simulink model "SS_elastico_SP"  (R2024b)
settings: Solver=VariableStepAuto  StartTime=0.0  StopTime=tsamplesimulink  RelTol=1e-3
undefined symbols (not defined in the file): Ac, Bcg, Cc, Dcg, Je, Jm, Kfd, Kfp, Kp, Kv, N, tm
settings Model: Creator=Isaac  LastModifiedBy=ruizh
settings SolverCC: AlgebraicLoopSolver=TrustRegion
settings DataIOCC: ReturnWorkspaceOutputs=off
settings DebuggingCC: UnconnectedInputMsg=warning  UnconnectedOutputMsg=warning  UnconnectedLineMsg=warning  ArithmeticOperatorsInVariantConditions=warning
settings ModelReferenceCC: EnableRefExpFcnMdlSchedulingChecks=on
settings SFSimCC: SimUseLocalCustomCode=off  CustomCodeUndefinedFunction=UseInterfaceOnly
settings RTWCC: RTWUseLocalCustomCode=off  GPUComputeCapability=3.5
settings CodeAppCC: StateflowObjectComments=on

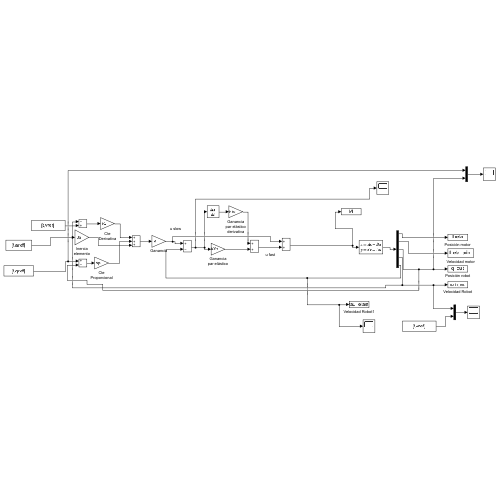
[thumbnail: Simulink's stored preview of the top-level diagram]
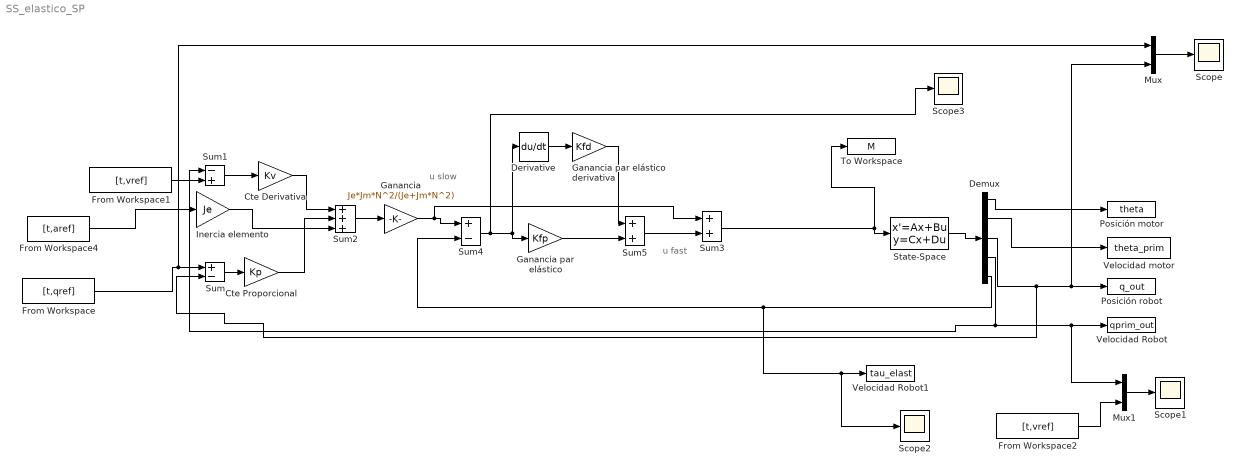
== system SS_elastico_SP ==
  note: u fast
  note: u slow
  Cte Derivativa : Gain  Gain=Kv  SaturateOnIntegerOverflow=on  OutDataTypeStr=Inherit: Same as input  ParamDataTypeStr=Inherit: Same as input
  Cte Proporcional : Gain  Gain=Kp  SaturateOnIntegerOverflow=on  OutDataTypeStr=Inherit: Same as input  ParamDataTypeStr=Inherit: Same as input
  Demux : Demux  Outputs=5
  Derivative : Derivative
  From Workspace : FromWorkspace  VariableName=[t,qref]  SampleTime=tm  ZeroCross=off
  From Workspace1 : FromWorkspace  VariableName=[t,vref]  SampleTime=tm  ZeroCross=off
  From Workspace2 : FromWorkspace  VariableName=[t,vref]  SampleTime=tm  ZeroCross=off
  From Workspace4 : FromWorkspace  VariableName=[t,aref]  SampleTime=tm  ZeroCross=off
  Ganancia : Gain  Gain=Je*Jm*N^2/(Je+Jm*N^2)  SaturateOnIntegerOverflow=on  OutDataTypeStr=Inherit: Same as input  ParamDataTypeStr=Inherit: Same as input
  Ganancia par elástico : Gain  Gain=Kfp  SaturateOnIntegerOverflow=on  OutDataTypeStr=Inherit: Same as input  ParamDataTypeStr=Inherit: Same as input
  Ganancia par elástico derivativa : Gain  Gain=Kfd  SaturateOnIntegerOverflow=on  OutDataTypeStr=Inherit: Same as input  ParamDataTypeStr=Inherit: Same as input
  Inercia elemento : Gain  Gain=Je  SaturateOnIntegerOverflow=on  OutDataTypeStr=Inherit: Same as input  ParamDataTypeStr=Inherit: Same as input
  Mux : Mux  Inputs=2
  Mux1 : Mux  Inputs=2
  Posición motor : ToWorkspace  VariableName=theta  SampleTime=tm
  Posición robot : ToWorkspace  VariableName=q_out  SampleTime=tm
  Scope{,1..3} (4 alike) : Scope
  State-Space : StateSpace  A=Ac  B=Bcg  C=Cc  D=Dcg  InitialCondition=0
  Sum : Sum  Inputs=+-  InputSameDT=on  SaturateOnIntegerOverflow=on  OutDataTypeStr=Inherit: Same as first input
  Sum1 : Sum  Inputs=-+  InputSameDT=on  SaturateOnIntegerOverflow=on  OutDataTypeStr=Inherit: Same as first input
  Sum2 : Sum  Inputs=+++  InputSameDT=on  SaturateOnIntegerOverflow=on  OutDataTypeStr=Inherit: Same as first input
  Sum3 : Sum  InputSameDT=on  SaturateOnIntegerOverflow=on  OutDataTypeStr=Inherit: Same as first input
  Sum4 : Sum  Inputs=+-  InputSameDT=on  SaturateOnIntegerOverflow=on  OutDataTypeStr=Inherit: Same as first input
  Sum5 : Sum  InputSameDT=on  SaturateOnIntegerOverflow=on  OutDataTypeStr=Inherit: Same as first input
  To Workspace : ToWorkspace  VariableName=M  SampleTime=tm
  Velocidad Robot : ToWorkspace  VariableName=qprim_out  SampleTime=tm
  Velocidad Robot1 : ToWorkspace  VariableName=tau_elast  SampleTime=tm
  Velocidad motor : ToWorkspace  VariableName=theta_prim  SampleTime=tm
  wires:
  Sum3/1 -> State-Space/1, To Workspace/1
  Demux/1 -> Posición motor/1
  Cte Derivativa/1 -> Sum2/1
  From Workspace/1 -> Sum/1, Mux/1
  Sum/1 -> Cte Proporcional/1
  Cte Proporcional/1 -> Sum2/2
  Demux/4 -> Sum1/1, Mux1/1, Velocidad Robot/1
  Sum1/1 -> Cte Derivativa/1
  From Workspace1/1 -> Sum1/2
  Demux/3 -> Sum/2, Mux/2, Posición robot/1
  Mux/1 -> Scope/1
  State-Space/1 -> Demux/1
  Demux/2 -> Velocidad motor/1
  Inercia elemento/1 -> Sum2/3
  From Workspace4/1 -> Inercia elemento/1
  Sum4/1 -> Scope3/1, Derivative/1, Ganancia par elástico/1
  Demux/5 -> Scope2/1, Velocidad Robot1/1, Sum4/2
  Mux1/1 -> Scope1/1
  From Workspace2/1 -> Mux1/2
  Derivative/1 -> Ganancia par elástico derivativa/1
  Sum2/1 -> Ganancia/1
  Ganancia/1 -> Sum3/1, Sum4/1
  Ganancia par elástico derivativa/1 -> Sum5/1
  Ganancia par elástico/1 -> Sum5/2
  Sum5/1 -> Sum3/2
